simulink model "gov_extended_2"  (R2020a)
settings: Solver=VariableStepAuto  StartTime=0.0  StopTime=10.0  RelTol=1e-3
values from neighbouring files (symbols this model uses):
  Kp = 10000    [main.m]
  sigma = 0.5    [main.m]
  target = 3500000    [main.m]
  Tf = 0.5    [main.m]
  Tg = 0.1    [main.m]
  To = 0.01    [main.m]
  Tp = 0.01    [main.m]
  tx = 0.4    [main.m]
  VAT = 0.07    [main.m]
settings Model: Creator=erlended  LastModifiedBy=erlended

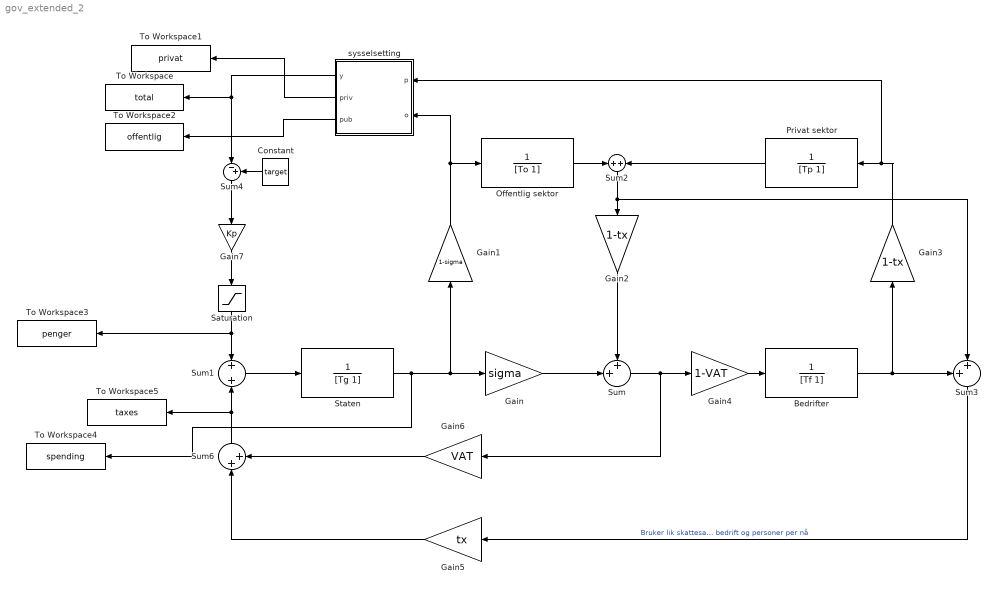
== system gov_extended_2 ==
  Bedrifter : TransferFcn  Denominator=[Tf 1]
  Constant : Constant  Value=target
  Gain : Gain  Gain=sigma
  Gain1 : Gain  Gain=1-sigma
  Gain2 : Gain  Gain=1-tx
  Gain3 : Gain  Gain=1-tx
  Gain4 : Gain  Gain=1-VAT
  Gain5 : Gain  Gain=tx
  Gain6 : Gain  Gain=VAT
  Gain7 : Gain  Gain=Kp
  Offentlig sektor : TransferFcn  Denominator=[To 1]
  Privat sektor : TransferFcn  Denominator=[Tp 1]
  Saturation : Saturate  UpperLimit=100000  LowerLimit=-100000
  Staten : TransferFcn  Denominator=[Tg 1]
  Sum : Sum  Inputs=++|
  Sum1 : Sum
  Sum2 : Sum  Inputs=+|+
  Sum3 : Sum  Inputs=++|
  Sum4 : Sum  Inputs=|-+
  Sum6 : Sum  Inputs=|++
  To Workspace : ToWorkspace  VariableName=total  SaveFormat=Timeseries  SampleTime=-1
  To Workspace1 : ToWorkspace  VariableName=privat  SaveFormat=Timeseries  SampleTime=-1
  To Workspace2 : ToWorkspace  VariableName=offentlig  SaveFormat=Timeseries  SampleTime=-1
  To Workspace3 : ToWorkspace  VariableName=penger  SaveFormat=Timeseries  SampleTime=-1
  To Workspace4 : ToWorkspace  VariableName=spending  SaveFormat=Timeseries  SampleTime=-1
  To Workspace5 : ToWorkspace  VariableName=taxes  SaveFormat=Timeseries  SampleTime=-1
  sysselsetting : MATLAB Function  TreatAsAtomicUnit=on
  wires:
  Staten/1 -> To Workspace4/1, Gain/1, Gain1/1
  Sum/1 -> Gain6/1, Gain4/1
  Gain1/1 -> Offentlig sektor/1, sysselsetting/2(o)
  Gain/1 -> Sum/2
  Privat sektor/1 -> Sum2/2
  Sum2/1 -> Gain2/1, Sum3/2
  Offentlig sektor/1 -> Sum2/1
  Sum1/1 -> Staten/1
  Gain4/1 -> Bedrifter/1
  sysselsetting/1(y) -> Sum4/1, To Workspace/1
  Bedrifter/1 -> Sum3/1, Gain3/1
  Sum3/1 -> Gain5/1  "Bruker lik skattesats på bedrift og personer per nå"
  Gain2/1 -> Sum/1
  Constant/1 -> Sum4/2
  Gain3/1 -> sysselsetting/1(p), Privat sektor/1
  sysselsetting/3(pub) -> To Workspace2/1
  sysselsetting/2(priv) -> To Workspace1/1
  Gain6/1 -> Sum6/2
  Gain5/1 -> Sum6/1
  Sum6/1 -> Sum1/2, To Workspace5/1
  Gain7/1 -> Saturation/1
  Sum4/1 -> Gain7/1
  Saturation/1 -> To Workspace3/1, Sum1/1

== matlab function gov_extended_2/sysselsetting ==
  data: p input; o input; y output; priv output; pub output
function  [y, priv, pub]= fcn(p, o)
salary = 0.5; 

priv = p/(salary);
pub = o/(salary);
u = priv + pub;

y = u;
